simulink model "soc_state_flow"  (R2016a)
settings: Solver=VariableStepAuto  StartTime=0.0  StopTime=1000  RelTol=1e-3
settings Model: Creator=hangyang  LastModifiedBy=hangyang

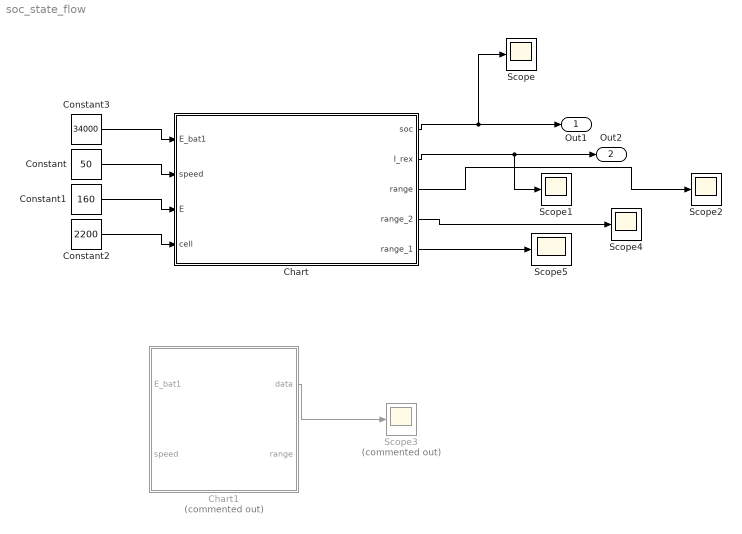
== system soc_state_flow ==
  Chart : Stateflow chart  TreatAsAtomicUnit=on
  Chart1 : Stateflow chart  Commented=on  TreatAsAtomicUnit=on
  Constant : Constant  Value=50
  Constant1 : Constant  Value=160
  Constant2 : Constant  Value=2200
  Constant3 : Constant  Value=34000
  Scope{,1..2,4..5} (5 alike) : Scope
  Scope3 : Scope  Commented=on
  Out1 : Outport
  Out2 : Outport  Port=2
  wires:
  Constant3/1 -> Chart/1(E_bat1)
  Constant/1 -> Chart/2(speed)
  Constant1/1 -> Chart/3(E)
  Constant2/1 -> Chart/4(cell)
  Chart/2(I_rex) -> Scope1/1, Out2/1
  Chart/3(range) -> Scope2/1
  Chart/1(soc) -> Scope/1, Out1/1
  Chart1/1(data) -> Scope3/1
  Chart/4(range_2) -> Scope4/1
  Chart/5(range_1) -> Scope5/1

== stateflow chart soc_state_flow/Chart1 ==
  (default) -> (junction 22) [order 2] : % for
  (junction 23) -> (junction 21) [order 1] : [i<101]
  (junction 21) -> (junction 24) : {soc=1*i;...
      |  rest=soc*E_bat1/100;...
      |  range_1=rest/E;...
      |  t=range_1/speed;...
      |  I_rex=3.1/t;...
      |  e_rex=1/(0.216+0.0479*I_rex);...
      |  E_rex=e_rex*cell;...
      |  range_2=E_rex/E;...
      |  range=range_1+range_2; }
  (default) -> (junction 8) [order 1] : % loop
  (junction 22) -> (junction 23) : {i=10;}
  (junction 9) -> (junction 7) [order 1] : [i<10]
  (junction 7) -> (junction 10) : {data=2*i;}
  (junction 8) -> (junction 9) : {i=0;}
  (junction 24) -> (junction 23) : {i=i+10;}
  (junction 23) -> (junction 25) [order 2]
  (junction 10) -> (junction 9) : {i = i + 1;}
  (junction 9) -> (junction 11) [order 2]
  data: data output; i local; E_bat1 input; speed input; range output; e_rex local; range_1 local; soc local; range_2 local; rest local; t local; I_rex local; E_rex local; E parameter

== stateflow chart soc_state_flow/Chart ==
  (default) -> (junction 52) : % while
  (junction 54) -> (junction 53) [order 1] : [range<250 && i<101]
  (junction 52) -> (junction 54) : {i=10;...
      | range=0;}
  (junction 53) -> (junction 55) : {soc=i;...
      |  rest=soc*E_bat1/100;...
      |  range_1=rest/E;...
      | range_bat1=E_bat1/E;...
      |  t=range_1/speed;...
      |  I_rex=3.1/t;...
      |  e_rex=1/(0.216+0.0479*I_rex)*cell;...
      |  range_2=e_rex/E;...
      |  range=range_bat1+range_2;...
      |  i=i+10;  }
  (junction 55) -> (junction 54)
  (junction 54) -> (junction 56) [order 2]
  data: E_bat1 input; speed input; E input; cell input; t local; e_rex local; E_rex local; rest local; soc output; I_rex output; range output; i local; range_2 output; range_1 output; range_bat1 local
